simulink model "wpt_plus_pfc_SS"  (R2022b)
settings: Solver=VariableStepAuto  StartTime=0.0  StopTime=0.1  RelTol=1e-3
undefined symbols (not defined in the file): Ion, Lithium
libraries: spsDiodeLib x9, spsVoltageMeasurementLib x7, spsCurrentMeasurementLib x6, spsSeriesRLCBranchLib x6, spsPowerPhasorLib x5, spsIGBTDiodeLib x4, spsPWMGeneratorDCDCLib x2, slpidlib x2, spsACVoltageSourceLib x1, spsBatteryLib x1, spsMutualInductanceLib x1, spsMosfetLib x1
settings Model: Creator=ahmed  LastModifiedBy=ahmed

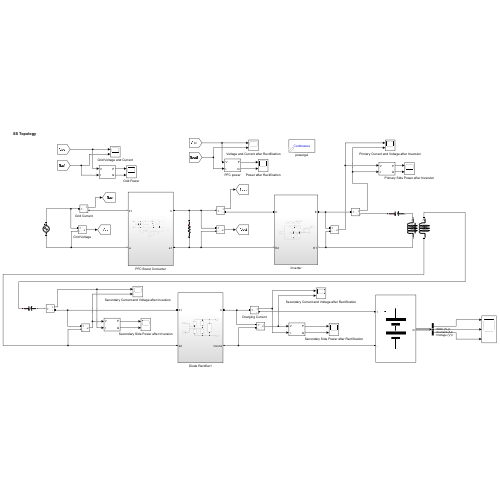
[thumbnail: Simulink's stored preview of the top-level diagram]
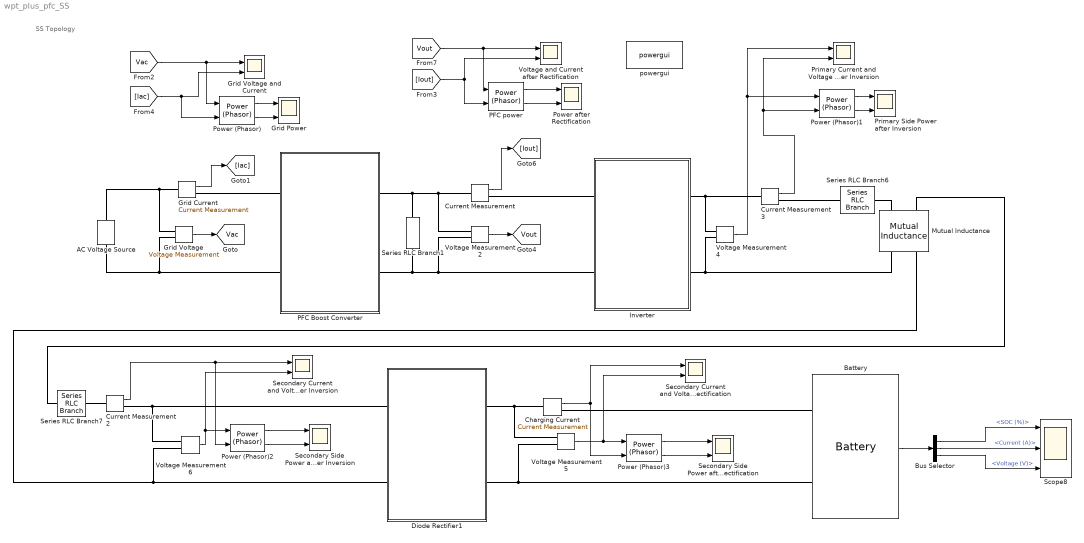
== system wpt_plus_pfc_SS ==
  note: SS Topology
  AC Voltage Source : spsACVoltageSourceLib/AC Voltage Source  Amplitude=325  Phase=0  Frequency=50  SampleTime=0  Measurements=None  BusType=swing  Pref=10e3  Qref=0  Qmin=-inf  Qmax=+inf
  Battery : spsBatteryLib/Battery  BatType=Lithium-Ion  ShowTempParam=off  ThermalPreset=no  ShowAgeParam=off  NomV=48  NomQ=150  SOC=90  Batt_Tr=0.1  PresetModel=on  MaxQ=150  MinV=36  FullV=55.8714  Dis_rate=65.2174  R=0.0032  Normal_OP=135.6522  expZone="[51.8585      7.36957]"  current=[6.5 13 32.5]  Units=Time  Tci=20  NomT=20  T2=-30  MaxQ2=4.8  FullV2=7.1  Normal_OP2=5.655  expZone2="[6.58           1]"  Rca=0.6  ti=2000  Dp=0  Neq0=0  Tsim=1e6  Ta1=25  Qeol=5.4*0.9  Reol=0.013333*1.2  Char_age=[2.3478, 3]  Dis_age=[2.3478, 10]  N1=1500  N2=10500  N3=1000  N4=1400  Ta2=45  N5=950
  Bus Selector : BusSelector  OutputSignals=SOC (%),Current (A),Voltage (V)
  Charging Current : spsCurrentMeasurementLib/Current Measurement  PhasorSimulation=off  OutputType=Complex  PSBequivalent=0
  Current Measurement : spsCurrentMeasurementLib/Current Measurement  PhasorSimulation=off  OutputType=Complex  PSBequivalent=0
  Current Measurement2 : spsCurrentMeasurementLib/Current Measurement  PhasorSimulation=off  OutputType=Complex  PSBequivalent=0
  Current Measurement3 : spsCurrentMeasurementLib/Current Measurement  PhasorSimulation=off  OutputType=Complex  PSBequivalent=0
  Diode Rectifier1 : Subsystem
  Grid Current : spsCurrentMeasurementLib/Current Measurement  PhasorSimulation=off  OutputType=Complex  PSBequivalent=0
  Grid Power : Scope  NumInputPorts=2
  Grid Voltage : spsVoltageMeasurementLib/Voltage Measurement  PhasorSimulation=off  OutputType=Complex  PSBequivalent=0
  Grid Voltage and Current : Scope  NumInputPorts=2
  Inverter : Subsystem
  Mutual Inductance : spsMutualInductanceLib/Mutual Inductance  LConnTagsString=a|b  RConnTagsString=A|B  TypeOfMutual=Two or three windings with equal mutual terms  NumberOfWindings=3  SelfImpedance1=[1e-3 137.804e-6]  SelfImpedance2=[ 1e-3 137.804e-6 ]  ThreeWindings=off  SelfImpedance3=[ 1.1 1.1e-03]  MutualImpedance=[0 36.236e-6 ]  InductanceMatrix="[1.0 0.9  0.9 ;  0.9 1.0  0.9;  0.9 0.9 1.0 ] * 1e-3"  ResistanceMatrix="[1.0 0.9  0.9 ;  0.9 1.0  0.9;  0.9 0.9 1.0 ]"  Measurements=None
  PFC Boost Converter : Subsystem
  PFC power : spsPowerPhasorLib/Power (Phasor)
  Power (Phasor){,1..3} (4 alike) : spsPowerPhasorLib/Power (Phasor)
  Power after Rectification : Scope  NumInputPorts=2
  Primary Current and Voltage after Inversion : Scope  NumInputPorts=2
  Primary Side Power after Inversion : Scope  NumInputPorts=2
  Scope8 : Scope  NumInputPorts=3
  Secondary Current and Voltage after Inversion : Scope  NumInputPorts=2
  Secondary Current and Voltage after Rectification : Scope  NumInputPorts=2
  Secondary Side Power after Inversion : Scope  NumInputPorts=2
  Secondary Side Power after Rectification : Scope  NumInputPorts=2
  Series RLC Branch1 : spsSeriesRLCBranchLib/Series RLC Branch  LConnTagsString=__new0  RConnTagsString=__new0  BranchType=R  Resistance=80  Inductance=1e-3  SetiL0=off  InitialCurrent=0  Capacitance=72.82e-9  Setx0=off  InitialVoltage=0  Measurements=None
  Series RLC Branch6 : spsSeriesRLCBranchLib/Series RLC Branch  LConnTagsString=__new0  RConnTagsString=__new0  BranchType=C  Resistance=1  Inductance=1e-3  SetiL0=off  InitialCurrent=0  Capacitance=39.093e-9  Setx0=off  InitialVoltage=0  Measurements=None
  Series RLC Branch7 : spsSeriesRLCBranchLib/Series RLC Branch  LConnTagsString=__new0  RConnTagsString=__new0  BranchType=C  Resistance=1  Inductance=1e-3  SetiL0=off  InitialCurrent=0  Capacitance=25.43e-9  Setx0=off  InitialVoltage=0  Measurements=None
  Voltage Measurement{2,4..6} (4 alike) : spsVoltageMeasurementLib/Voltage Measurement  PhasorSimulation=off  OutputType=Complex  PSBequivalent=0
  Voltage and Current after Rectification : Scope  NumInputPorts=2
  powergui : spspowerguiLib/powergui  Priority=1  SimulationMode=Continuous  SampleTime=1e-6  frequency=60  Iterations=50  frequencyindice=0  Pbase=100e6  ErrMax=1e-4  UnitsV=kV  UnitsW=MW  buscounter=0  FunctionMessages=off  echomessages=off  EnableUseOfTLC=off  CurrentSourceSwitches=off  DisableSnubberDevices=off  DisableRonSwitches=off  DisableVfSwitches=off  DisplayEquations=off  AutomaticDiscreteSolvers=off  SolverType=Tustin/Backward Euler (TBE)  Interpol=off  ExternalGateDelay=off  methode=off  Ts=100  x0status=blocks  SPID=on  SwTol=0  HookPort=off  NonlinearTolerance=1e-4  nMaxIteration=100  ContinueOnMaxIteration=off  RestoreLinks=warning  ResistiveCurrentMeasurement=off  Frange=[0:2:500]  Ylog=off  Xlog=on  ShowGrid=off  save=off  variable=ZData  structure=0  ZoomFFT=off  StartTime=0.0  cycles=1  DisplayStyle=1  fundamental=60  FreqAxis=off  MaxFrequency=1000  frequencyindicesteady=1  RmsSteady=1  display=off
  tag scope: Vac=global, Vout=global
  wires:
  Current Measurement2/1 -> Secondary Current and Voltage after Inversion/1, Power (Phasor)2/2
  Charging Current/1 -> Secondary Current and Voltage after Rectification/1, Power (Phasor)3/2
  [Iac] -> Grid Voltage and Current/2, Power (Phasor)/2
  Voltage Measurement5/1 -> Secondary Current and Voltage after Rectification/2, Power (Phasor)3/1
  [Iout] -> Voltage and Current after Rectification/2, PFC power/2
  Power (Phasor)2/1 -> Secondary Side Power after Inversion/1
  [Vout] -> Voltage and Current after Rectification/1, PFC power/1
  Current Measurement3/1 -> Primary Current and Voltage after Inversion/2, Power (Phasor)1/2
  Power (Phasor)2/2 -> Secondary Side Power after Inversion/2
  Power (Phasor)1/1 -> Primary Side Power after Inversion/1
  Voltage Measurement4/1 -> Primary Current and Voltage after Inversion/1, Power (Phasor)1/1
  Power (Phasor)3/1 -> Secondary Side Power after Rectification/1
  Voltage Measurement2/1 -> [Vout]
  [Vac] -> Grid Voltage and Current/1, Power (Phasor)/1
  Power (Phasor)3/2 -> Secondary Side Power after Rectification/2
  Voltage Measurement6/1 -> Secondary Current and Voltage after Inversion/2, Power (Phasor)2/1
  Bus Selector/3 -> Scope8/3  "<Voltage (V)>"
  Power (Phasor)/2 -> Grid Power/2
  Battery/1 -> Bus Selector/1
  Grid Voltage/1 -> [Vac]
  Power (Phasor)1/2 -> Primary Side Power after Inversion/2
  Current Measurement/1 -> [Iout]
  PFC power/1 -> Power after Rectification/1
  Bus Selector/2 -> Scope8/2  "<Current (A)>"
  Power (Phasor)/1 -> Grid Power/1
  Bus Selector/1 -> Scope8/1  "<SOC (%)>"
  PFC power/2 -> Power after Rectification/2
  Grid Current/1 -> [Iac]
  connections:
  PFC Boost Converter/RConn1 -- Series RLC Branch1/LConn1 -- Voltage Measurement2/LConn1 -- Current Measurement/LConn1
  Voltage Measurement6/LConn2 -- Diode Rectifier1/LConn2 -- Mutual Inductance/RConn2
  Grid Voltage/LConn1 -- AC Voltage Source/RConn1 -- Grid Current/LConn1
  Diode Rectifier1/RConn1 -- Charging Current/LConn1 -- Voltage Measurement5/LConn1
  AC Voltage Source/LConn1 -- Grid Voltage/LConn2 -- PFC Boost Converter/LConn2
  Current Measurement2/RConn1 -- Diode Rectifier1/LConn1 -- Voltage Measurement6/LConn1
  Inverter/RConn1 -- Voltage Measurement4/LConn1 -- Current Measurement3/LConn1
  Voltage Measurement5/LConn2 -- Diode Rectifier1/RConn2 -- Battery/LConn2
  Inverter/LConn2 -- Voltage Measurement2/LConn2 -- PFC Boost Converter/RConn2 -- Series RLC Branch1/RConn1
  Voltage Measurement4/LConn2 -- Mutual Inductance/RConn1 -- Inverter/RConn2
  Current Measurement3/RConn1 -- Series RLC Branch6/LConn1
  Current Measurement2/LConn1 -- Series RLC Branch7/RConn1
  Battery/LConn1 -- Charging Current/RConn1
  PFC Boost Converter/LConn1 -- Grid Current/RConn1
  Mutual Inductance/LConn1 -- Series RLC Branch6/RConn1
  Current Measurement/RConn1 -- Inverter/LConn1
  Mutual Inductance/LConn2 -- Series RLC Branch7/LConn1

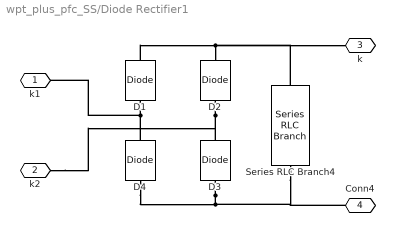
== system wpt_plus_pfc_SS/Diode Rectifier1 ==
  D{1..4} (4 alike) : spsDiodeLib/Diode  Ron=0.001  Lon=0  Vf=0.8  IC=0  UseSnubber=0  Rs=500  Cs=250e-9  Measurements=off
  Series RLC Branch4 : spsSeriesRLCBranchLib/Series RLC Branch  LConnTagsString=__new0  RConnTagsString=__new0  BranchType=C  Resistance=1  Inductance=1e-3  SetiL0=off  InitialCurrent=0  Capacitance=100e-6  Setx0=off  InitialVoltage=0  Measurements=None
  k1 : PMIOPort  Side=Left
  k2 : PMIOPort  Port=2  Side=Left
  k : PMIOPort  Port=3  Side=Right
  Conn4 : PMIOPort  Port=4  Side=Right
  connections:
  D3/LConn1 -- D4/LConn1 -- Series RLC Branch4/RConn1 -- Conn4/RConn1
  D2/LConn1 -- D3/RConn1 -- k2/RConn1
  D2/RConn1 -- D1/RConn1 -- Series RLC Branch4/LConn1 -- k/RConn1
  D4/RConn1 -- D1/LConn1 -- k1/RConn1

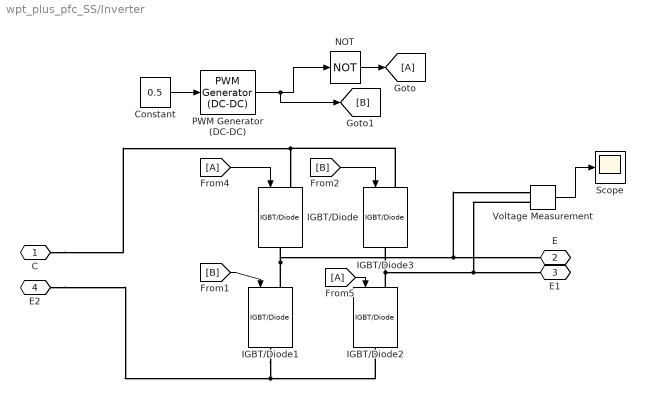
== system wpt_plus_pfc_SS/Inverter ==
  Constant : Constant  Value=0.5
  From4 : From
  From5 : From
  Goto : Goto
  IGBT/Diode{,1..3} (4 alike) : spsIGBTDiodeLib/IGBT//Diode  Ron=1e-3  Rs=1e5  Cs=inf  Measurements=off
  NOT : Logic  Operator=NOT  IconShape=distinctive  AllPortsSameDT=off  OutDataTypeStr=boolean
  PWM Generator (DC-DC) : spsPWMGeneratorDCDCLib/PWM Generator (DC-DC)  Fsw=85000  Ts=0
  Scope : Scope
  Voltage Measurement : spsVoltageMeasurementLib/Voltage Measurement  PhasorSimulation=off  OutputType=Complex  PSBequivalent=0
  C : PMIOPort  Side=Left
  E : PMIOPort  Port=2  Side=Right
  E1 : PMIOPort  Port=3  Side=Right
  E2 : PMIOPort  Port=4  Side=Left
  wires:
  NOT/1 -> Goto/1
  From5/1 -> IGBT/Diode2/1
  Constant/1 -> PWM Generator (DC-DC)/1
  [B] -> IGBT/Diode1/1
  From4/1 -> IGBT/Diode/1
  PWM Generator (DC-DC)/1 -> [B], NOT/1
  [B] -> IGBT/Diode3/1
  Voltage Measurement/1 -> Scope/1
  connections:
  IGBT/Diode2/LConn1 -- IGBT/Diode3/RConn1 -- Voltage Measurement/LConn2 -- E1/RConn1
  IGBT/Diode1/RConn1 -- E2/RConn1 -- IGBT/Diode2/RConn1
  IGBT/Diode3/LConn1 -- C/RConn1 -- IGBT/Diode/LConn1
  IGBT/Diode1/LConn1 -- IGBT/Diode/RConn1 -- Voltage Measurement/LConn1 -- E/RConn1

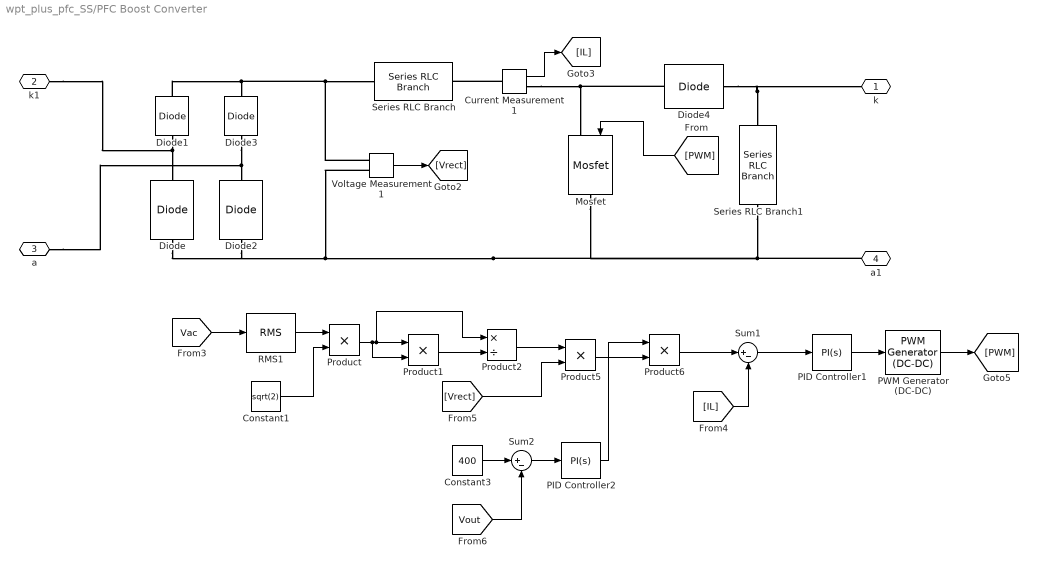
== system wpt_plus_pfc_SS/PFC Boost Converter ==
  Constant1 : Constant  Value=sqrt(2)
  Constant3 : Constant  Value=400
  Current Measurement1 : spsCurrentMeasurementLib/Current Measurement  PhasorSimulation=off  OutputType=Complex  PSBequivalent=0
  Diode{,1..4} (5 alike) : spsDiodeLib/Diode  Ron=0.001  Lon=0  Vf=0.8  IC=0  UseSnubber=0  Rs=500  Cs=250e-9  Measurements=off
  Mosfet : spsMosfetLib/Mosfet  Ron=0.1  Lon=0  Rd=0.01  Vfd=0  IC=0  Rs=1e5  Cs=inf  Measurements=off
  PID Controller1 : slpidlib/PID Controller  Controller=PI  Form=Parallel  TimeDomain=Continuous-time  UseExternalTs=off  SampleTime=-1  IntegratorMethod=Forward Euler  FilterMethod=Forward Euler  ControllerParametersSource=internal  P=2000  I=0.25  UseKiTs=off  D=0  N=100  UseFilter=on  TunerSelectOption=Transfer Function Based (PID Tuner App)  InitialConditionSource=internal  InitialConditionForIntegrator=0  InitialConditionForFilter=0  DifferentiatorICPrevScaledInput=0  ExternalReset=none  TrackingMode=off  Kt=1  LimitOutput=on  SatLimitsSource=internal  UpperSaturationLimit=0.95  LowerSaturationLimit=0  LinearizeAsGain=on  AntiWindupMode=none  Kb=1  LimitIntegrator=off  UpperIntegratorSaturationLimit=inf  LowerIntegratorSaturationLimit=-inf  POutMin=[]  POutMax=[]  IOutMin=[]  IOutMax=[]  DOutMin=[]  DOutMax=[]  NOutMin=[]  NOutMax=[]  SumOutMin=[]  SumOutMax=[]  SaturationOutMin=[]  SaturationOutMax=[]  PParamMin=[]  PParamMax=[]  IParamMin=[]  IParamMax=[]  DParamMin=[]  DParamMax=[]  NParamMin=[]  NParamMax=[]  KbParamMin=[]  KbParamMax=[]  KtParamMin=[]  KtParamMax=[]  KbOutMin=[]  KbOutMax=[]  KtOutMin=[]  KtOutMax=[]  IntegratorOutMin=[]  IntegratorOutMax=[]  FilterOutMin=[]  FilterOutMax=[]  SumI1OutMin=[]  SumI1OutMax=[]  SumI2OutMin=[]  SumI2OutMax=[]  SumI3OutMin=[]  SumI3OutMax=[]  SumI4OutMin=[]  SumI4OutMax=[]  SumDOutMin=[]  SumDOutMax=[]  DifferentiatorOutMin=[]  DifferentiatorOutMax=[]  FilterDiffOutCoefMin=[]  FilterDiffOutCoefMax=[]  ReciprocalOutMin=[]  ReciprocalOutMax=[]  SumDenOutMin=[]  SumDenOutMax=[]  SumNumOutMin=[]  SumNumOutMax=[]  DivideOutMin=[]  DivideOutMax=[]  UdiffTsProdOutMin=[]  UdiffTsProdOutMax=[]  NTsProdOutMin=[]  NTsProdOutMax=[]  UintegralTsProdOutMin=[]  UintegralTsProdOutMax=[]  UngainTsProdOutMin=[]  UngainTsProdOutMax=[]  ClampingZeroOutDataTypeStr=Inherit: Inherit via back propagation  ClampingZeroOutMin=[]  ClampingZeroOutMax=[]  FilterDenConstantOutDataTypeStr=Inherit: Inherit via back propagation  FilterDenConstantOutMin=[]  FilterDenConstantOutMax=[]  PCopyOutDataTypeStr=Inherit: Inherit via back propagation  PCopyOutMin=[]  PCopyOutMax=[]  NCopyOutDataTypeStr=Inherit: Inherit via back propagation  NCopyOutMin=[]  NCopyOutMax=[]  IntegratorContinuousStateAttributes=''  IntegratorStateMustResolveToSignalObject=off  IntegratorRTWStateStorageClass=Auto  FilterContinuousStateAttributes=''  FilterStateMustResolveToSignalObject=off  FilterRTWStateStorageClass=Auto  ParallelPVariant=InternalParameters  IdealPVariant=Disabled  IVariant=InternalParameters  DVariant=Disabled  IntegratorVariant=Continuous  SatVariant=Enabled  AWVariant=Passthrough  PCopyVariant=Disabled  TRVariant=Disabled  FdbkBlocksVariant=Forward  IdealPFdbkVariant=Disabled  SatFdbkVariant=Disabled  DerivativeFilterVariant=Disabled  NVariant=Disabled  NCopyVariant=Disabled_SignalSpec  FilterICVariant=Disabled  IntegratorICVariant=InternalICs  ExternalResetVariant=Disabled  TRSumVariant=Passthrough  SumFdbkVariant=Disabled  SumVariant=Sum_PI  TsampFilterVariant=InternalTs  TsampNgainVariant=Passthrough  TsampIntegralVariant=Passthrough  ExternalSaturationOutDataTypeStr=Inherit: Same as second input
  PID Controller2 : slpidlib/PID Controller  Controller=PI  Form=Parallel  TimeDomain=Continuous-time  UseExternalTs=off  SampleTime=-1  IntegratorMethod=Forward Euler  FilterMethod=Forward Euler  ControllerParametersSource=internal  P=0.25  I=35  UseKiTs=off  D=0  N=100  UseFilter=on  TunerSelectOption=Transfer Function Based (PID Tuner App)  InitialConditionSource=internal  InitialConditionForIntegrator=0  InitialConditionForFilter=0  DifferentiatorICPrevScaledInput=0  ExternalReset=none  TrackingMode=off  Kt=1  LimitOutput=off  SatLimitsSource=internal  UpperSaturationLimit=inf  LowerSaturationLimit=-inf  LinearizeAsGain=on  AntiWindupMode=none  Kb=1  LimitIntegrator=off  UpperIntegratorSaturationLimit=inf  LowerIntegratorSaturationLimit=-inf  POutMin=[]  POutMax=[]  IOutMin=[]  IOutMax=[]  DOutMin=[]  DOutMax=[]  NOutMin=[]  NOutMax=[]  SumOutMin=[]  SumOutMax=[]  SaturationOutMin=[]  SaturationOutMax=[]  PParamMin=[]  PParamMax=[]  IParamMin=[]  IParamMax=[]  DParamMin=[]  DParamMax=[]  NParamMin=[]  NParamMax=[]  KbParamMin=[]  KbParamMax=[]  KtParamMin=[]  KtParamMax=[]  KbOutMin=[]  KbOutMax=[]  KtOutMin=[]  KtOutMax=[]  IntegratorOutMin=[]  IntegratorOutMax=[]  FilterOutMin=[]  FilterOutMax=[]  SumI1OutMin=[]  SumI1OutMax=[]  SumI2OutMin=[]  SumI2OutMax=[]  SumI3OutMin=[]  SumI3OutMax=[]  SumI4OutMin=[]  SumI4OutMax=[]  SumDOutMin=[]  SumDOutMax=[]  DifferentiatorOutMin=[]  DifferentiatorOutMax=[]  FilterDiffOutCoefMin=[]  FilterDiffOutCoefMax=[]  ReciprocalOutMin=[]  ReciprocalOutMax=[]  SumDenOutMin=[]  SumDenOutMax=[]  SumNumOutMin=[]  SumNumOutMax=[]  DivideOutMin=[]  DivideOutMax=[]  UdiffTsProdOutMin=[]  UdiffTsProdOutMax=[]  NTsProdOutMin=[]  NTsProdOutMax=[]  UintegralTsProdOutMin=[]  UintegralTsProdOutMax=[]  UngainTsProdOutMin=[]  UngainTsProdOutMax=[]  ClampingZeroOutDataTypeStr=Inherit: Inherit via back propagation  ClampingZeroOutMin=[]  ClampingZeroOutMax=[]  FilterDenConstantOutDataTypeStr=Inherit: Inherit via back propagation  FilterDenConstantOutMin=[]  FilterDenConstantOutMax=[]  PCopyOutDataTypeStr=Inherit: Inherit via back propagation  PCopyOutMin=[]  PCopyOutMax=[]  NCopyOutDataTypeStr=Inherit: Inherit via back propagation  NCopyOutMin=[]  NCopyOutMax=[]  IntegratorContinuousStateAttributes=''  IntegratorStateMustResolveToSignalObject=off  IntegratorRTWStateStorageClass=Auto  FilterContinuousStateAttributes=''  FilterStateMustResolveToSignalObject=off  FilterRTWStateStorageClass=Auto  ParallelPVariant=InternalParameters  IdealPVariant=Disabled  IVariant=InternalParameters  DVariant=Disabled  IntegratorVariant=Continuous  SatVariant=Disabled  AWVariant=Passthrough  PCopyVariant=Disabled  TRVariant=Disabled  FdbkBlocksVariant=Forward  IdealPFdbkVariant=Disabled  SatFdbkVariant=Disabled  DerivativeFilterVariant=Disabled  NVariant=Disabled  NCopyVariant=Disabled_SignalSpec  FilterICVariant=Disabled  IntegratorICVariant=InternalICs  ExternalResetVariant=Disabled  TRSumVariant=Passthrough  SumFdbkVariant=Disabled  SumVariant=Sum_PI  TsampFilterVariant=InternalTs  TsampNgainVariant=Passthrough  TsampIntegralVariant=Passthrough  ExternalSaturationOutDataTypeStr=Inherit: Same as second input
  PWM Generator (DC-DC) : spsPWMGeneratorDCDCLib/PWM Generator (DC-DC)  Fsw=65000  Ts=1e-6
  Product{,1,5..6} (4 alike) : Product
  Product2 : Product  Inputs=*/
  RMS1 : spsRMSLib/RMS  TrueRMS=on  Freq=50  RMSInit=230  Ts=0
  Series RLC Branch : spsSeriesRLCBranchLib/Series RLC Branch  LConnTagsString=__new0  RConnTagsString=__new0  BranchType=L  Resistance=1  Inductance=0.3e-3  SetiL0=off  InitialCurrent=0  Capacitance=1e-6  Setx0=off  InitialVoltage=0  Measurements=None
  Series RLC Branch1 : spsSeriesRLCBranchLib/Series RLC Branch  LConnTagsString=__new0  RConnTagsString=__new0  BranchType=C  Resistance=1  Inductance=1e-3  SetiL0=off  InitialCurrent=0  Capacitance=2000e-6  Setx0=off  InitialVoltage=0  Measurements=None
  Sum1 : Sum  Inputs=|+-
  Sum2 : Sum  Inputs=|+-
  Voltage Measurement1 : spsVoltageMeasurementLib/Voltage Measurement  PhasorSimulation=off  OutputType=Complex  PSBequivalent=0
  k : PMIOPort  Side=Right
  k1 : PMIOPort  Port=2  Side=Left
  a : PMIOPort  Port=3  Side=Left
  a1 : PMIOPort  Port=4  Side=Right
  wires:
  Voltage Measurement1/1 -> [Vrect]
  [IL] -> Sum1/2
  PWM Generator (DC-DC)/1 -> [PWM]
  Current Measurement1/1 -> [IL]
  Sum1/1 -> PID Controller1/1
  PID Controller1/1 -> PWM Generator (DC-DC)/1
  [PWM] -> Mosfet/1
  Product6/1 -> Sum1/1
  Product2/1 -> Product5/1
  Product5/1 -> Product6/2
  Product/1 -> Product2/1, Product1/1, Product1/2
  [Vrect] -> Product5/2
  Constant1/1 -> Product/2
  [Vout] -> Sum2/2
  Constant3/1 -> Sum2/1
  PID Controller2/1 -> Product6/1
  Product1/1 -> Product2/2
  Sum2/1 -> PID Controller2/1
  RMS1/1 -> Product/1
  [Vac] -> RMS1/1
  connections:
  k1/RConn1 -- Diode1/LConn1 -- Diode/RConn1
  Diode4/RConn1 -- Series RLC Branch1/LConn1 -- k/RConn1
  Voltage Measurement1/LConn1 -- Diode1/RConn1 -- Diode3/RConn1 -- Series RLC Branch/LConn1
  a1/RConn1 -- Series RLC Branch1/RConn1 -- Mosfet/RConn1 -- Diode2/LConn1 -- Diode/LConn1 -- Voltage Measurement1/LConn2
  Current Measurement1/RConn1 -- Mosfet/LConn1 -- Diode4/LConn1
  Diode3/LConn1 -- Diode2/RConn1 -- a/RConn1
  Current Measurement1/LConn1 -- Series RLC Branch/RConn1
